simulink model "sim_model"  (Simulink 8.0)
settings: Solver=ode45  StartTime=0.0  StopTime=10.0  RelTol=1e-3
libraries: fmu_me_lib x1
settings Model: Creator=Tin Rabuzin  LastModifiedBy=Tin Rabuzin
settings DebuggingCC: AlgebraicLoopMsg=error  SolverPrmCheckMsg=none

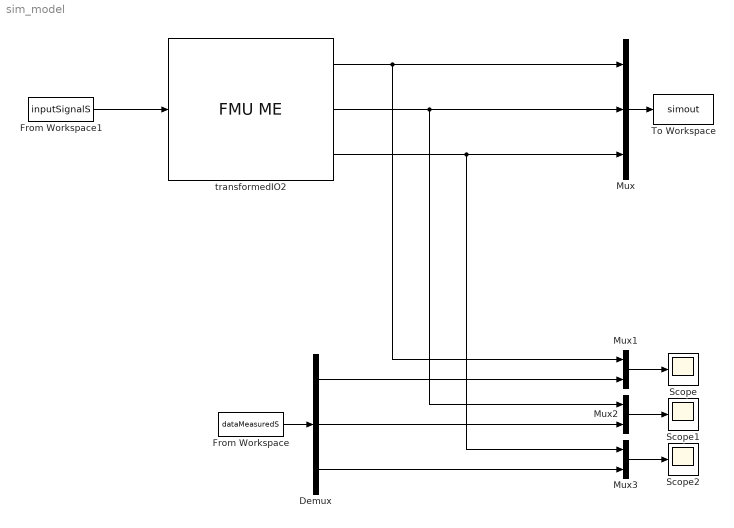
== system sim_model ==
  Demux : Demux  Outputs=3
  From Workspace : FromWorkspace  VariableName=dataMeasuredS  SampleTime=0
  From Workspace1 : FromWorkspace  VariableName=inputSignalS  SampleTime=0
  Mux : Mux  Inputs=3
  Mux1 : Mux  Inputs=2
  Mux2 : Mux  Inputs=2
  Mux3 : Mux  Inputs=2
  Scope : Scope
  Scope1 : Scope
  Scope2 : Scope
      settings: YMin=0.399  YMax=0.411  SaveName=ScopeData2
  To Workspace : ToWorkspace  VariableName=simout  SampleTime=-1  SaveFormat=Structure With Time
  transformedIO2 : fmu_me_lib/FMU ME  Description=Simulates an FMU for Model Exchange 1.0 or Model Exchange 2.0.
  wires:
  transformedIO2/1 -> Mux1/1, Mux/1
  transformedIO2/2 -> Mux2/1, Mux/2
  transformedIO2/3 -> Mux3/1, Mux/3
  Mux1/1 -> Scope/1
  Mux2/1 -> Scope1/1
  Mux3/1 -> Scope2/1
  Demux/1 -> Mux1/2
  Demux/2 -> Mux2/2
  Demux/3 -> Mux3/2
  From Workspace/1 -> Demux/1
  From Workspace1/1 -> transformedIO2/1
  Mux/1 -> To Workspace/1
